simulink model "model_benchmark_sim1"  (R2018a)
settings: Solver=VariableStepAuto  StartTime=0.0  StopTime=100  RelTol=1e-3
values from neighbouring files (symbols this model uses):
  ae1 = model_identified.Parameters(3).Value    [model_benchmark_init.m]    (also in workspace.mat = 1.36231449822)
  ae2 = model_identified.Parameters(4).Value    [model_benchmark_init.m]    (also in workspace.mat = -0.378717172069)
  at = model_identified.Parameters(7).Value    [model_benchmark_init.m]    (also in workspace.mat = -0.463804529993)
  be = model_identified.Parameters(6).Value    [model_benchmark_init.m]    (also in workspace.mat = 0.116311837295)
  bl = model_identified.Parameters(2).Value    [model_benchmark_init.m]    (also in workspace.mat = 0.103160863637)
  bt = model_identified.Parameters(9).Value    [model_benchmark_init.m]    (also in workspace.mat = 0.962119048974)
  ce = model_identified.Parameters(5).Value    [model_benchmark_init.m]    (also in workspace.mat = 0.04469700002)
  cl = model_identified.Parameters(1).Value    [model_benchmark_init.m]    (also in workspace.mat = 0.202457747385)
  ct = model_identified.Parameters(8).Value    [model_benchmark_init.m]    (also in workspace.mat = 0.00762763482449)
  par_ctrl = struct    [model_benchmark_init.m]    (also in workspace.mat = )
  par_id = struct    [model_benchmark_init.m]    (also in workspace.mat = )
  x0 = [0; 0; 0.1745; 0; -0.1047; 0]    [model_benchmark_init.m]    (also in model_benchmark_ode45.m = [0; 0; 0; 0; 0.1; 0]; workspace.mat = [0 0 0.1745 0 -0.1047 0])
libraries: simulink_extras x1
settings Model: Creator=obrusvit  LastModifiedBy=obrusvit

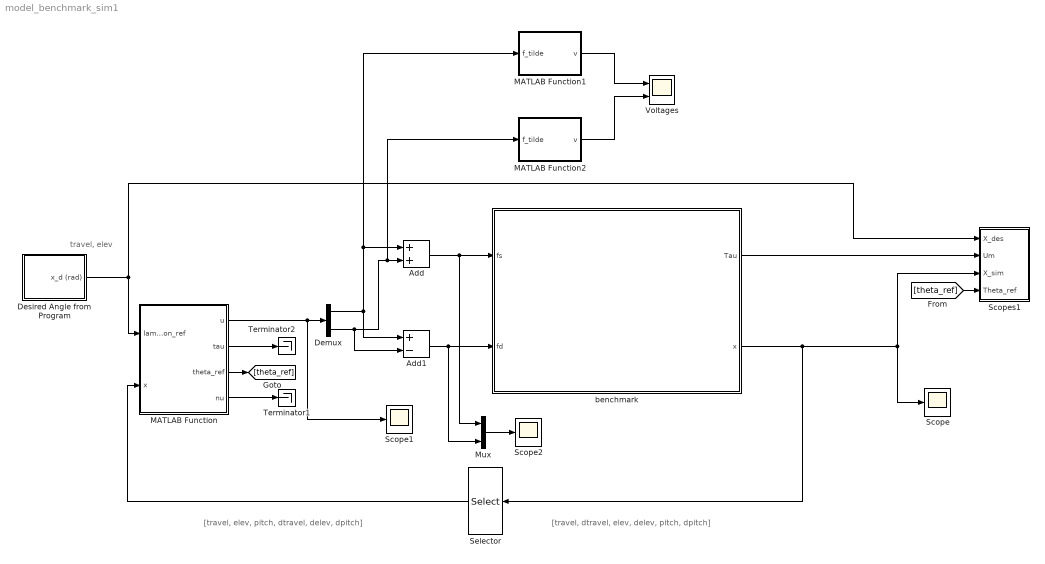
== system model_benchmark_sim1 ==
  note: travel, elev
  note: [travel, dtravel, elev, delev, pitch, dpitch]
  note: [travel, elev, pitch, dtravel, delev, dpitch]
  Add : Sum
  Add1 : Sum  Inputs=+-
  Demux : Demux  Outputs=2
  Desired Angle from Program : Subsystem
  MATLAB Function : MATLAB Function  TreatAsAtomicUnit=on
  MATLAB Function1 : MATLAB Function  TreatAsAtomicUnit=on
  MATLAB Function2 : MATLAB Function  TreatAsAtomicUnit=on
  Mux : Mux  Inputs=2
  Scope : Scope
  Scope1 : Scope
  Scope2 : Scope
  Scopes1 : Subsystem
  Selector : Selector  InputPortWidth=6  IndexOptions=Index vector (dialog)  Indices=[1 3 5 2 4 6]  OutputSizes=1
  Terminator1 : Terminator
  Terminator2 : Terminator
  "Voltages " : Scope  NumInputPorts=2
  benchmark : Subsystem
  wires:
  Desired Angle from Program/1(x_d (rad)) -> MATLAB Function/1(lambda_epsilon_ref), Scopes1/1(X_des)
  MATLAB Function/1(u) -> Scope1/1, Demux/1
  benchmark/1(Tau) -> Scopes1/2("Um ")
  Add/1 -> benchmark/1("fs "), Mux/1
  Add1/1 -> benchmark/2("fd "), Mux/2
  benchmark/2(x) -> Selector/1, Scopes1/3(X_sim), Scope/1
  Mux/1 -> Scope2/1
  Selector/1 -> MATLAB Function/2(x)
  MATLAB Function/3(theta_ref) -> [theta_ref]
  MATLAB Function/4(nu) -> Terminator1/1
  MATLAB Function/2(tau) -> Terminator2/1
  [theta_ref] -> Scopes1/4(Theta_ref)
  MATLAB Function1/1(v) -> "Voltages "/1
  Demux/2 -> Add1/2, MATLAB Function2/1(f_tilde), Add/2
  Demux/1 -> Add1/1, MATLAB Function1/1(f_tilde), Add/1
  MATLAB Function2/1(v) -> "Voltages "/2

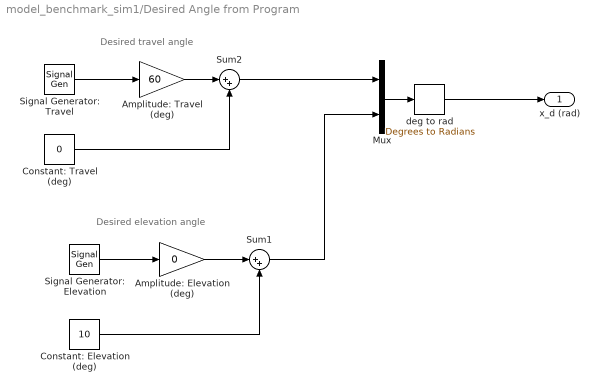
== system model_benchmark_sim1/Desired Angle from Program ==
  note: Desired elevation angle
  note: Desired travel angle
  Amplitude: Elevation (deg) : Gain  Gain=0
  Amplitude: Travel (deg) : Gain  Gain=60
  Constant: Elevation (deg) : Constant  Value=10
  Constant: Travel (deg) : Constant  Value=0
  Mux : Mux  Inputs=2
  Signal Generator: Elevation : SignalGenerator  WaveForm=square  Frequency=0.04
  Signal Generator: Travel : SignalGenerator  WaveForm=square  Frequency=0.01
  Sum1 : Sum  Inputs=|++
  Sum2 : Sum  Inputs=|++
  deg to rad : simulink_extras/Transformations/Degrees to Radians
  x_d (rad) : Outport
  wires:
  Mux/1 -> deg to rad/1
  Constant: Elevation (deg)/1 -> Sum1/2
  Amplitude: Elevation (deg)/1 -> Sum1/1
  Signal Generator: Elevation/1 -> Amplitude: Elevation (deg)/1
  Constant: Travel (deg)/1 -> Sum2/2
  Amplitude: Travel (deg)/1 -> Sum2/1
  Signal Generator: Travel/1 -> Amplitude: Travel (deg)/1
  Sum1/1 -> Mux/2
  deg to rad/1 -> x_d (rad)/1
  Sum2/1 -> Mux/1

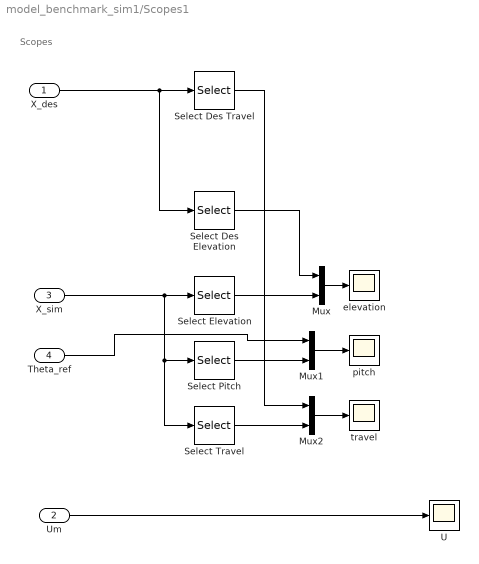
== system model_benchmark_sim1/Scopes1 ==
  note: Scopes
  X_des : Inport
  "Um " : Inport  Port=2
  X_sim : Inport  Port=3
  Theta_ref : Inport  Port=4
  Mux : Mux  Inputs=2
  Mux1 : Mux  Inputs=2
  Mux2 : Mux  Inputs=2
  Select Des Elevation : Selector  InputPortWidth=2  IndexOptions=Index vector (dialog)  Indices=2  OutputSizes=1
  Select Des Travel : Selector  InputPortWidth=2  IndexOptions=Index vector (dialog)  Indices=1  OutputSizes=1
  Select Elevation : Selector  InputPortWidth=6  IndexOptions=Index vector (dialog)  Indices=3  OutputSizes=1
  Select Pitch : Selector  InputPortWidth=6  IndexOptions=Index vector (dialog)  Indices=5  OutputSizes=1
  Select Travel : Selector  InputPortWidth=6  IndexOptions=Index vector (dialog)  Indices=1  OutputSizes=1
  U : Scope
  "elevation " : Scope
  pitch : Scope
  travel : Scope
  wires:
  Mux/1 -> "elevation "/1
  Mux1/1 -> pitch/1
  "Um "/1 -> U/1
  X_sim/1 -> Select Elevation/1, Select Pitch/1, Select Travel/1
  Mux2/1 -> travel/1
  Select Elevation/1 -> Mux/2
  Select Pitch/1 -> Mux1/2
  Select Travel/1 -> Mux2/2
  X_des/1 -> Select Des Elevation/1, Select Des Travel/1
  Select Des Elevation/1 -> Mux/1
  Select Des Travel/1 -> Mux2/1
  Theta_ref/1 -> Mux1/1

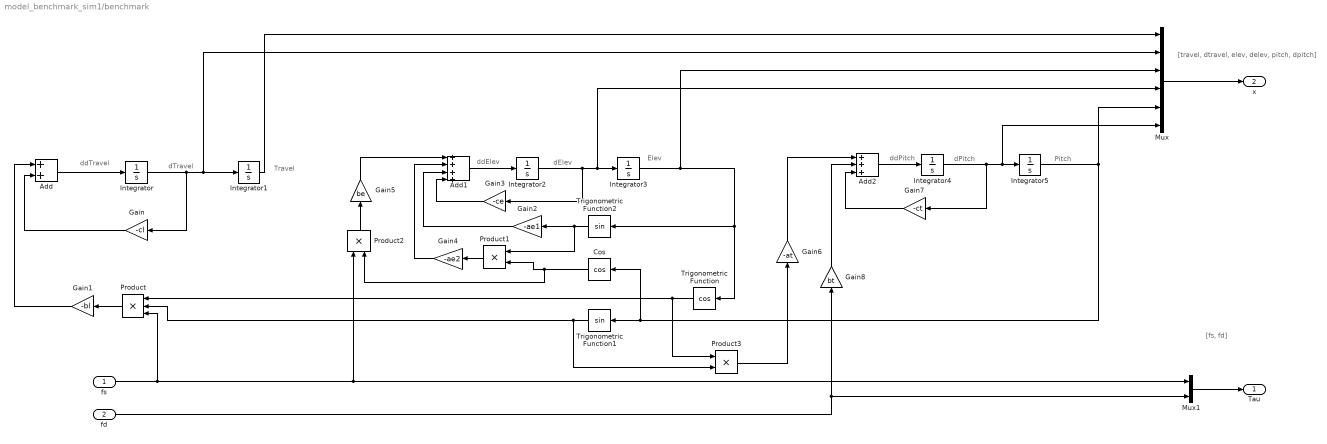
== system model_benchmark_sim1/benchmark ==
  note: [travel, dtravel, elev, delev, pitch, dpitch]
  note: Pitch
  note: dPitch
  note: ddPitch
  note: Elev
  note: dElev
  note: ddElev
  note: Travel
  note: dTravel
  note: ddTravel
  note: [fs, fd]
  "fs " : Inport
  "fd " : Inport  Port=2
  Add : Sum
  Add1 : Sum  Inputs=++++
  Add2 : Sum  Inputs=+++
  Cos : Trigonometry  Operator=cos
  Gain : Gain  Gain=-cl
  Gain1 : Gain  Gain=-bl
  Gain2 : Gain  Gain=-ae1
  Gain3 : Gain  Gain=-ce
  Gain4 : Gain  Gain=-ae2
  Gain5 : Gain  Gain=be
  Gain6 : Gain  Gain=-at
  Gain7 : Gain  Gain=-ct
  Gain8 : Gain  Gain=bt
  Integrator : Integrator  InitialCondition=x0(2)
  Integrator1 : Integrator  InitialCondition=x0(1)
  Integrator2 : Integrator  InitialCondition=x0(4)
  Integrator3 : Integrator  InitialCondition=x0(3)
  Integrator4 : Integrator  InitialCondition=x0(6)
  Integrator5 : Integrator  InitialCondition=x0(5)
  Mux : Mux  Inputs=6
  Mux1 : Mux  Inputs=2
  Product : Product  Inputs=3
  Product1 : Product
  Product2 : Product
  Product3 : Product
  Trigonometric Function : Trigonometry  Operator=cos
  Trigonometric Function1 : Trigonometry
  Trigonometric Function2 : Trigonometry
  Tau : Outport
  x : Outport  Port=2
  wires:
  Gain5/1 -> Add1/1
  Product/1 -> Gain1/1
  Product2/1 -> Gain5/1
  "fd "/1 -> Mux1/2, Gain8/1
  Trigonometric Function/1 -> Product3/1, Product/1
  Product3/1 -> Gain6/1
  Gain7/1 -> Add2/3
  Cos/1 -> Product2/2, Product1/2
  Gain4/1 -> Add1/2
  Gain2/1 -> Add1/3
  Mux/1 -> x/1
  Gain8/1 -> Add2/2
  Add2/1 -> Integrator4/1
  Gain6/1 -> Add2/1
  Integrator1/1 -> Mux/1
  Gain1/1 -> Add/1
  Integrator3/1 -> Mux/3, Trigonometric Function2/1, Trigonometric Function/1
  Integrator2/1 -> Gain3/1, Mux/4, Integrator3/1
  Product1/1 -> Gain4/1
  Gain3/1 -> Add1/4
  Integrator4/1 -> Gain7/1, Mux/6, Integrator5/1
  Integrator/1 -> Gain/1, Integrator1/1, Mux/2
  Gain/1 -> Add/2
  Add1/1 -> Integrator2/1
  Integrator5/1 -> Cos/1, Trigonometric Function1/1, Mux/5
  Trigonometric Function2/1 -> Product1/1, Gain2/1
  Trigonometric Function1/1 -> Product3/2, Product/2
  "fs "/1 -> Mux1/1, Product2/1, Product/3
  Add/1 -> Integrator/1
  Mux1/1 -> Tau/1

== matlab function model_benchmark_sim1/MATLAB Function1 ==
  data: f_tilde input; v output; par parameter
function v = fcn(f_tilde, par)

v = scaled_force_2_voltage(f_tilde, par.exp.scaled_f_2_v_par, par.exp.scaled_f_2_v_ths);

== matlab function model_benchmark_sim1/MATLAB Function ==
  data: lambda_epsilon_ref input; x input; u output; tau output; theta_ref output; nu output; par_id parameter; par_ctrl parameter
function [u, tau, theta_ref, nu] = fcn(lambda_epsilon_ref, x, par_id, par_ctrl)

T = diag([-par_id.bl*cos(x(2)), par_id.be, par_id.bt]);

g_bar = [0;...
         sin(x(2))*(par_id.ae1+par_id.ae2*cos(x(3)))*0.95;...
         par_id.at*cos(x(2))*sin(x(3))];

R_bar = diag([par_id.cl, par_id.ce, par_id.ct]);
                    

nu = [0;0;0];

nu(1:2) = pinv(T(1:2, 1:2)) * ( g_bar(1:2)   -   par_ctrl.Omega(1:2,1:2)^2 * (x(1:2)-lambda_epsilon_ref)   +   (R_bar(1:2,1:2) - par_ctrl.Xi(1:2,1:2)) * x(4:5) );
nu(1) = nu(1) - 0.12;

theta_ref = atan2( nu(1), nu(2) );

if abs(x(2)<deg2rad(1))
    theta_ref = 0;
end


nu(3)   = pinv(T(3, 3)) * (g_bar(3)   -   par_ctrl.Omega(3,3)^2 * (x(3)-theta_ref)   +   (R_bar(3,3) - par_ctrl.Xi(3,3)) * x(6));

B = [sin(x(3)) 0;...
      cos(x(3)) 0;...
     0          1];
tau = B'*nu;

u = [1/2  1/2;...
     1/2 -1/2]* tau;

== matlab function model_benchmark_sim1/MATLAB Function2 ==
  data: f_tilde input; v output; par parameter
function v = fcn(f_tilde, par)

v = scaled_force_2_voltage(f_tilde, par.exp.scaled_f_2_v_par, par.exp.scaled_f_2_v_ths);
